simulink model "lqr_stabilization"  (R2018a)
settings: Solver=VariableStepAuto  StartTime=0.0  StopTime=5.0  RelTol=1e-3
libraries: simulink x1
Description:
  | LQR state-feedback control
  | 
  | Copyright 2023-2024 University of Ulsan, ECSL.
settings Model: Creator=Kim  LastModifiedBy=Kim

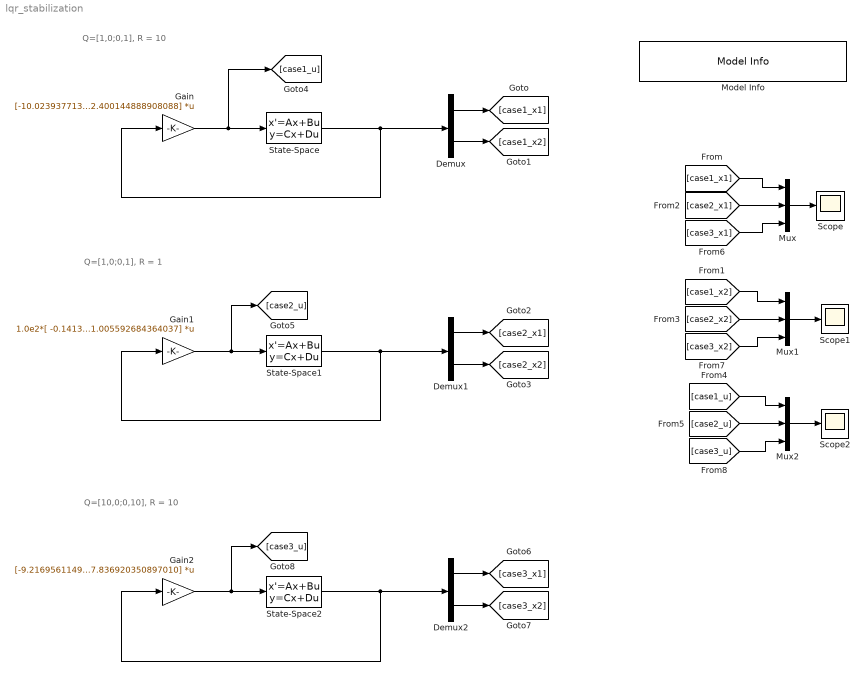
== system lqr_stabilization ==
  note: Q=[1,0;0,1], R = 1
  note: Q=[1,0;0,1], R = 10
  note: Q=[10,0;0,10], R = 10
  Demux : Demux  Outputs=2
  Demux1 : Demux  Outputs=2
  Demux2 : Demux  Outputs=2
  Gain : Gain  Gain=[-10.023937713572201 -52.400144888908088]  Multiplication=Matrix(K*u)
  Gain1 : Gain  Gain="1.0e2*[ -0.141393319563934  -1.005592684364037]"  Multiplication=Matrix(K*u)
  Gain2 : Gain  Gain=[-9.216956114942937 -47.836920350897010]  Multiplication=Matrix(K*u)
  Model Info : simulink/Model-Wide Utilities/Model Info  Frame=on  DisplayStringWithTags=|  HorizontalTextAlignment=Center  LeftAlignmentValue=0.5
      | Model Info
      | 
      | LQR state-feedback control systems
  Mux : Mux  Inputs=3
  Mux1 : Mux  Inputs=3
  Mux2 : Mux  Inputs=3
  Scope : Scope
  Scope1 : Scope
  Scope2 : Scope
  State-Space : StateSpace  A=[ 1, -2 ; 1, 4]  B=[1; 0.1]  C=[1, 0; 0, 1]  D=[0; 0]  InitialCondition=[1,-1]
  State-Space1 : StateSpace  A=[ 1, -2 ; 1, 4]  B=[1; 0.1]  C=[1, 0; 0, 1]  D=[0; 0]  InitialCondition=[1,-1]
  State-Space2 : StateSpace  A=[ 1, -2 ; 1, 4]  B=[1; 0.1]  C=[1, 0; 0, 1]  D=[0; 0]  InitialCondition=[1,-1]
  wires:
  State-Space/1 -> Gain/1, Demux/1
  Gain/1 -> [case1_u], State-Space/1
  Gain1/1 -> [case2_u], State-Space1/1
  State-Space1/1 -> Demux1/1, Gain1/1
  Demux/1 -> [case1_x1]
  Demux/2 -> [case1_x2]
  Demux1/2 -> [case2_x2]
  Demux1/1 -> [case2_x1]
  Mux/1 -> Scope/1
  [case1_x1] -> Mux/1
  [case2_x1] -> Mux/2
  Mux1/1 -> Scope1/1
  [case2_u] -> Mux2/2
  [case1_u] -> Mux2/1
  Mux2/1 -> Scope2/1
  [case2_x2] -> Mux1/2
  [case1_x2] -> Mux1/1
  Demux2/1 -> [case3_x1]
  Demux2/2 -> [case3_x2]
  State-Space2/1 -> Gain2/1, Demux2/1
  Gain2/1 -> State-Space2/1, [case3_u]
  [case3_x2] -> Mux1/3
  [case3_x1] -> Mux/3
  [case3_u] -> Mux2/3
